simulink model "Transicao"  (R2015b)
settings: Solver=FixedStepAuto  StartTime=0  StopTime=120  FixedStep=sampleTime  RelTol=1e-3
InitFcn:
  | sampleTime = 0.01;
  | Ktd = 0.0526/1000;
  | Kdd = 0.0526/1000;
  | Lb = [0.27 0.27 0.27 0.27];
  | LbAssimetrico  = [0.27 0.27 0.18 0.36];
  | LbTeste  = [0.27 0.27 0.18 0.36];
  | Ixx = 0.0754483;
  | Iyy = 0.13642;
  | Izz = 0.2043333;
  | 
  | IXYZ = [Ixx 0 0; 0 Iyy 0; 0 0 Izz];
  | 
  | areaLateral = [0.0114398 0 0; 0 0.09533687 0; 0 0 0.33];
  | 
  | areaAsa = 0.243;
  | areaProfundor = 0.051;
  | densidadeAr = 1.2;
  | cdArrastoParasita = 1.5;
  | clAviao = 0.825;
  | cdAviao = 0.0743;
  | g = 9.8;
  | massa = 3;
  | velCruzeiro = 15;
  | 
  | inicioTransicao = 40;
  | inicioDesativaAtivacao = 80;
  | 
  | global kroll
  | global kpitch
  | global kyaw
  | 
  | global kx
  | global ky
  | global kz
  | 
  | %Voo em cruzeiro
  | global ku
  | global kzprof
  | global kpitchprof
undefined symbols (not defined in the file or in its folder): DiscIntNeverNeededParam, kpitch, kpitchprof, kroll, ku, kx, kyaw, kz, kzprof
libraries: simulink x17, aerolibwind2 x1
(part 1 of 2)
settings Model: Creator=Avell-G1711  LastModifiedBy=Avell-G1711

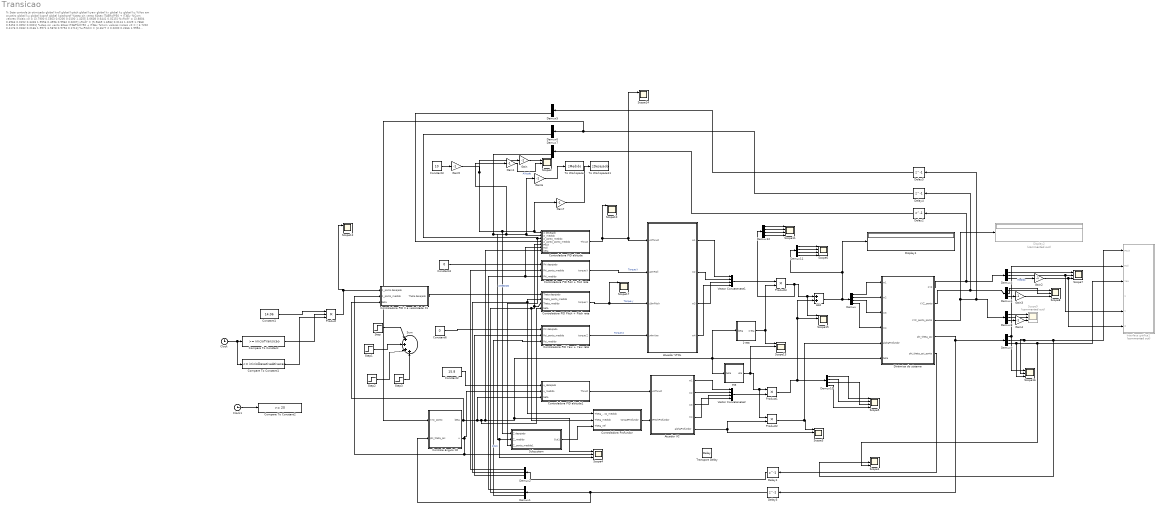
== system Transicao ==
  note: % Seta controle já otimizado
      | global kroll
      | global kpitch
      | global kyaw
      | global kx
      | global ky
      | global kz
      |
      | %Voo em cruzeiro
      | global ku
      | global kzprof
      | global kpitchprof
      |
      | %step sin vento 60sec ITAERoll*50 + ITAEy
      | %Com valores iniciais x0 = [3.7900    0.1663    0.0200    0.0100    1.4255    3.0608    0.6441    0.0215]
      | %xRollY = [3.8804    0.3963    0.0152    0.3328    1.9556    0.4596 0.9962    0.0207]
      | xRollY = [5.5669    1.6582    0.0113    1.2229    1.7868    0.5453    0.0052    0.0001]
      |
      | %step sin vento 60sec ITAEPitch*50 + ITAEx
      | %Com valores iniciais x0 = [ 3.7202    0.4176    0.0182    0.2166    1.9971    3.5878    0.9794    0.1711]
      | %xPitchX = [3.3677    2    0.0200    0.2366    1.9994    0.5776    0.9994    0.0200]
      | %xPitchX = [4.4401    2.8617    0.0114    1.9908    1.9994    4.5196    0.9994    0.0146]
      | %ISExPitchX = [4.0959    0.7473    0.0117    0.0115    2.6735    5.2103    1.9231    0.0301]
      |
      | % VTOL
      | xPitchX = [3.4125    1.4194    0.0110    0.2067    1.8694    3.1439    1.6099    0.0001]
      |
      | %QUASEVTOL mudou apenas o velocidade X pra ajudar na desaceleração
      | xPitchX1 = [3.4125    1.4194    0.0110    0.2067    1.8694    0.6    1.6099    0.0001]
      | %Beta até pi/2.5
      | %xPitchX2 = [8.0000    4.9999    0.0003    2.0000     1.9994    0.5776    0.9994    0.0200]
      |
      | %Beta depois de pi/2.5 (só pra pitch
      | xPitchX2 = [7.1864    4.9121    0.1706    1.1068   1.9994    3.1439    1.6099    0.0001]
      |
      | %Durante VC, foda-se a velocidade em VTOL
      | xPitchX3 = [7.1864    4.9121    0.1706    1.1068   1.9994   0    0    0]
      |
      |
      | %xPitchX2 = [7.1864    4.9121    0.1706    1.1068   1.9994    0    0    0]
      |
      |
      | %beta = 0
      | %xZ = [1.0370    7.9791    1.4905    0.0191    1.2406]
      | xZ = [1.1656    8   3.6063  0   0.6026]
      | %beta = alto
      | xZ2 = [0.1    20    2.5    0    0.5]
      |
      |
      | %Velocidade transição
      | %xu = [3.9966    0.0200    0.0000]
      | %xu = [7.9999    0.0123    1.9988]
      | %xu = [7.9999    0.0123    1.9995]
      | %xu = [15.0000    0.0000    2.2014]
      |
      | %xu 90 graus
      |
      | %xu = [7.9980    0.0015    0.9654]
      | %xu em transicao
      | xu = [10    0.0044    0.0201] %<pi/2.5
      | xu2 = [10    0.0044      5] %>pi/2.5
      |
      |
      |
      | %beta 90 graus
      | %xpitchz = [7.9805    0.0011    0.0210    1.9925    0.0002    0.0360    0.3908    0.0000    0.0000   0.0231    0.0014    0.0263]
      |
      | xpitchz = [9.9883    0.0015    0.0210    7.9750    0.0001    0.0000    0.5    0.0001    0.0000   0.04    0.0051    0.03]
      |
      |
      | kroll.kp = xRollY(1);
      | kroll.kp_ponto = xRollY(2);
      | kroll.kd_ponto = xRollY(3);
      | kroll.ki_ponto = xRollY(4);
      |
      | kpitch.betas = [0   pi/8];
      | kpitch.kp = [xPitchX(1) xPitchX2(1)];
      | kpitch.kp_ponto = [xPitchX(2) xPitchX2(2)];
      | kpitch.kd_ponto = [xPitchX(3) xPitchX2(3)];
      | kpitch.ki_ponto = [xPitchX(4) xPitchX2(4)];
      |
      | kyaw.kp = 2;
      | kyaw.kp_ponto = 2;
      | kyaw.kd_ponto = 0.0134;
      | kyaw.ki_ponto = 2;
      |
      | kx.betas = [pi/3  pi/2.5];
      | kx.kp = xPitchX(5);
      | kx.kp_ponto = [xPitchX1(6)   xPitchX3(6)];
      | kx.kd_ponto =  [xPitchX1(7)   xPitchX3(7)];
      | kx.ki_ponto =  [xPitchX1(8)   xPitchX3(8)];
      |
      | ky.kp = xRollY(5);
      | ky.kp_ponto = xRollY(6);
      | ky.kd_ponto = xRollY(7);
      | ky.ki_ponto = xRollY(8);
      |
      | kz.betas = [0   pi/6];
      | kz.kp = [xZ(1)  xZ2(1)];
      | kz.kp_ponto = [xZ(2)  xZ2(2)];
      | kz.kp_ponto_ponto = [xZ(3)  xZ2(3)];
      | kz.kd_ponto_ponto = [xZ(4)  xZ2(4)];
      | kz.ki_ponto_ponto = [xZ(5)  xZ2(5)];
      |
      | ku.betas = [pi/2.5  pi/2]
      | ku.kp = [xu(1)  xu2(1)];
      | ku.kd = [xu(2)  xu2(2)];
      | ku.ki = [xu(3)  xu2(3)];
      |
      |
      |
      | kpitchprof.kp = xpitchz(1);
      | kpitchprof.kd = xpitchz(2);
      | kpitchprof.ki = xpitchz(3);
      | kpitchprof.kp_ponto = xpitchz(4);
      | kpitchprof.kd_ponto = xpitchz(5);
      | kpitchprof.ki_ponto = xpitchz(6);
      |
      | kzprof.kp = xpitchz(7);
      | kzprof.kd = xpitchz(8);
      | kzprof.ki = xpitchz(9);
      | kzprof.kp_ponto = xpitchz(10);
      | kzprof.kd_ponto = xpitchz(11);
      | kzprof.ki_ponto = xpitchz(12);
      |
      |
      | % global eta
      | % global beta
      | % beta = pi/12;
      | % eta = beta/(pi/2)
      | a=10;
  1-eta : Subsystem
  Add : Sum
  Atuador VC : Subsystem
  Atuador VTOL : Subsystem
  Clock : Clock
  Clock1 : Clock
  Compare To Constant : simulink/Logic and Bit Operations/Compare To Constant  relop=>=  const=inicioTransicao  OutDataTypeStr=boolean
  Compare To Constant1 : simulink/Logic and Bit Operations/Compare To Constant  relop=<=  const=inicioDesativaAtivacao  OutDataTypeStr=boolean
  Compare To Constant2 : simulink/Logic and Bit Operations/Compare To Constant  relop=>=  const=20  OutDataTypeStr=boolean
  Constant1 : Constant  Value=14.06
  Constant2 : Constant  Value=15.8
  Constant3 : Constant  Value=10
  Constant4 : Constant  Value=0
  Constant6 : Constant  Value=0
  Controladora PID Pitch + Pitch rate : Subsystem
  Controladora PID Roll + Roll rate : Subsystem
  Controladora PID X e velocidade X1 : Subsystem
  Controladora PID Yaw + Yaw rate : Subsystem
  Controladora PID altitude : Subsystem
  Controladora PID altitude1 : Subsystem
  Controladora Profundor : Subsystem
  Controle ângulo tilt : Subsystem
  Delay{1..5} (5 alike) : Delay  DelayLength=1  InitialCondition=[0 0 0]
  Demux{,10..12} (4 alike) : Demux
  Demux{1..9} (9 alike) : Demux  Outputs=3
  Dinâmica do sistema : Subsystem
  Display1 : Display
  Display2 : Display  Commented=on
  Gain{,1..7} (8 alike) : Gain  Gain=-1
  Interface gráfica1 : Subsystem  Commented=on  AncestorBlock=vampLib/Interface gráfica
  Product : Product  Inputs=3
  Product1 : Product
  Product2 : Product
  Product3 : Product
  Scope{1..2,4,7..8,12,14,16} (8 alike) : Scope  NumInputPorts=3
  Scope{3,5..6,10..11,13,15,17} (8 alike) : Scope  NumInputPorts=4
  Scope9 : Scope  Commented=on  NumInputPorts=3
  Step : Step  Time=0  After=10  SampleTime=0
  Step1 : Step  Time=20  After=10  SampleTime=0
  Step2 : Step  Time=50  After=-20  SampleTime=0
  Step3 : Step  Time=80  After=10  SampleTime=0
  Subsystem : Subsystem
  Sum : Sum  Inputs=|++++
  To Workspace : ToWorkspace  VariableName=zMedido  SaveFormat=Timeseries  SampleTime=-1
  To Workspace11 : ToWorkspace  VariableName=zDesejado  SaveFormat=Timeseries  SampleTime=-1
  Transport Delay : TransportDelay  DelayTime=20
  Vector Concatenate1 : Concatenate  NumInputs=4
  Vector Concatenate2 : Concatenate  NumInputs=4
  eta : Subsystem
  wires:
  Demux3/1 -> Scope7/1
  Demux3/2 -> Interface gráfica1/5(Y), Scope7/2
  Demux3/3 -> Gain2/1  "Medido"
  Demux4/1 -> Scope8/1
  Demux4/2 -> Scope8/2
  Demux4/3 -> Gain3/1
  Dinâmica do sistema/2(XYZ_ponto) -> Delay4/1, Demux4/1
  Dinâmica do sistema/4(phi_theta_psi) -> Demux9/1, Delay3/1
  Dinâmica do sistema/5(phi_theta_psi_ponto) -> Delay1/1
  Delay1/1 -> Demux2/1
  Demux2/1 -> Controladora PID Roll + Roll rate/2(Phi_ponto_medido)
  Demux2/2 -> Controladora Profundor/1(Theta_ponto_medido), Controladora PID Pitch + Pitch rate/2(Theta_ponto_medido)
  Demux2/3 -> Controladora PID Yaw + Yaw rate/2(Psi_ponto_medido)
  Demux1/1 -> Controladora PID altitude/6(Roll), Controladora PID Roll + Roll rate/3(Phi_medido)
  Demux1/2 -> Controladora Profundor/2(Theta_medido), Controladora PID altitude/5(Pitch), Controladora PID Pitch + Pitch rate/3(Theta_medido)  "Pitch"
  Controladora PID Roll + Roll rate/1(torque X) -> Atuador VTOL/2(u2mRoll)  "Torque X"
  Controladora PID Pitch + Pitch rate/1(torque Y) -> Scope17/1, Atuador VTOL/3(u3mPitch)  "Torque y"
  Controladora PID Yaw + Yaw rate/1(torque Z) -> Atuador VTOL/4(u4mYaw)  "Torque Z"
  Demux7/3 -> Scope4/3, Subsystem/2(Z_medido), Controladora PID altitude/2(Z_medido), Gain6/1, Gain1/1  "ZMEDIDO"
  Dinâmica do sistema/1(XYZ) -> Delay2/1, Demux3/1
  Delay5/1 -> Demux5/1
  Delay4/1 -> Controle ângulo tilt/1(XYZ_ponto), Demux6/1
  Delay2/1 -> Demux7/1
  Demux5/3 -> Controladora PID altitude/4(Z_ponto_ponto_medido)
  Demux6/3 -> Subsystem/3(Z_ponto_medido1), Controladora PID altitude/3(Z_ponto_medido)
  Demux8/1 -> Scope9/1
  Demux8/2 -> Scope9/2
  Demux8/3 -> Gain4/1
  Dinâmica do sistema/3(XYZ_ponto_ponto) -> Display2/1, Demux8/1, Delay5/1
  Gain/1 -> Scope2/1
  Gain1/1 -> Scope2/2  "Alitude"
  Gain2/1 -> Interface gráfica1/6(Z), Scope7/3
  Gain3/1 -> Scope8/3
  Gain4/1 -> Scope9/3
  Demux9/3 -> Scope16/3, Scope1/3, Interface gráfica1/3(Yaw)
  Controladora PID altitude/1(Thrust) -> Scope10/1, Scope14/1, Atuador VTOL/1(u1Thrust)
  Demux1/3 -> Controladora PID Yaw + Yaw rate/3(Psi_medido)
  Gain5/1 -> Subsystem/1(Z desejado), Gain7/1, Controladora PID altitude/1(Z desejado), Gain/1
  Controladora PID altitude1/1(Thrust) -> Atuador VC/1(u1Thrust)
  Atuador VTOL/1(w1) -> Vector Concatenate1/1
  Atuador VTOL/2(w2) -> Vector Concatenate1/2
  Atuador VTOL/3(w3) -> Vector Concatenate1/3
  Atuador VTOL/4(w4) -> Vector Concatenate1/4
  Atuador VC/1(w1) -> Vector Concatenate2/1
  Atuador VC/2(w2) -> Vector Concatenate2/2
  Atuador VC/3(w3) -> Vector Concatenate2/3
  Atuador VC/4(w4) -> Vector Concatenate2/4
  Vector Concatenate2/1 -> Product1/2
  eta/1(eta) -> Scope13/2, Product2/1, Product1/1
  Demux/1 -> Dinâmica do sistema/1(w1)
  Demux/2 -> Dinâmica do sistema/2(w2)
  Demux/3 -> Dinâmica do sistema/3(w3)
  Demux/4 -> Dinâmica do sistema/4(w4)
  Atuador VC/5(alphaProfundor) -> Product2/2, Scope3/2
  Product2/1 -> Dinâmica do sistema/5(alphaProfundor), Scope3/1
  Controle ângulo tilt/1(beta) -> Controladora PID altitude1/3(beta), Controladora PID Pitch + Pitch rate/4(beta), Controladora PID altitude/7(beta), Scope4/1, 1-eta/1(beta), eta/1(beta), Dinâmica do sistema/6(beta), Controladora PID X e velocidade X1/3(beta)
  Controle ângulo tilt/2(u) -> Controladora PID altitude1/2(u_medido), Scope4/2, Controladora PID X e velocidade X1/2(X_ponto_medido)
  Delay3/1 -> Controle ângulo tilt/2(phi_theta_psi), Demux1/1
  Constant4/1 -> Controladora PID Roll + Roll rate/1(Phi desejado)
  Controladora PID X e velocidade X1/1(Theta desejado) -> Controladora PID Pitch + Pitch rate/1(Theta desejado)
  Constant6/1 -> Controladora PID Yaw + Yaw rate/1(Psi desejado)
  Controladora Profundor/1(torqueProfundor) -> Atuador VC/2(tPitchProfundor)
  Demux9/1 -> Scope16/1, Interface gráfica1/2(Roll)
  Subsystem/1(Out1) -> Controladora Profundor/3(Theta_ref)
  1-eta/1(1-eta) -> Product3/2, Scope13/1
  Demux10/1 -> Scope5/1
  Demux10/2 -> Scope5/2
  Demux10/3 -> Scope5/3
  Demux10/4 -> Scope5/4
  Product1/1 -> Add/2, Scope15/2, Demux10/1
  Demux11/1 -> Scope6/1
  Demux11/2 -> Scope6/2
  Demux11/3 -> Scope6/3
  Demux11/4 -> Scope6/4
  Demux12/1 -> Scope11/1
  Demux12/2 -> Scope11/2
  Demux12/3 -> Scope11/3
  Demux12/4 -> Scope11/4
  Product3/1 -> Demux12/1, Scope15/1, Add/1
  Vector Concatenate1/1 -> Product3/1
  Add/1 -> Display1/1, Demux11/1, Demux/1
  Demux9/2 -> Scope16/2, Scope1/2, Interface gráfica1/1(Pitch)
  Clock/1 -> Compare To Constant1/1, Compare To Constant/1
  Compare To Constant/1 -> Product/2
  Compare To Constant1/1 -> Product/3
  Constant1/1 -> Product/1
  Product/1 -> Scope12/1, Controladora PID X e velocidade X1/1(X_ponto desejado)
  Step/1 -> Sum/1
  Step1/1 -> Sum/2
  Step2/1 -> Sum/3
  Step3/1 -> Sum/4
  Clock1/1 -> Compare To Constant2/1
  Gain6/1 -> To Workspace/1
  Gain7/1 -> To Workspace11/1
  Constant2/1 -> Controladora PID altitude1/1(u_desejado)
  Constant3/1 -> Gain5/1

== system Transicao/1-eta ==
  beta : Inport
  Constant : Constant  Value=pi/2
  Constant1 : Constant
  Divide : Product  Inputs=*/
  Sum : Sum  Inputs=|+-
  1-eta : Outport
  wires:
  beta/1 -> Divide/1
  Divide/1 -> Sum/2
  Constant/1 -> Divide/2
  Constant1/1 -> Sum/1
  Sum/1 -> 1-eta/1

== system Transicao/Atuador VC ==
  u1Thrust : Inport
  tPitchProfundor : Inport  Port=2
  Kdd1 : Constant  Value=Kdd
  Ktd1 : Constant  Value=Ktd
  Motor mixer : MATLAB Function  TreatAsAtomicUnit=on
  ib1 : Constant  Value=Lb
  w1 : Outport
  w2 : Outport  Port=2
  w3 : Outport  Port=3
  w4 : Outport  Port=4
  alphaProfundor : Outport  Port=5
  wires:
  tPitchProfundor/1 -> Motor mixer/2(u3mPitch)
  ib1/1 -> Motor mixer/5(lb)
  Motor mixer/2(w2) -> w2/1
  Motor mixer/1(w1) -> w1/1
  u1Thrust/1 -> Motor mixer/1(u1thrust)
  Motor mixer/3(w3) -> w3/1
  Motor mixer/4(w4) -> w4/1
  Ktd1/1 -> Motor mixer/3(ktd)
  Kdd1/1 -> Motor mixer/4(kdd)
  Motor mixer/5(alphaProfundor) -> alphaProfundor/1

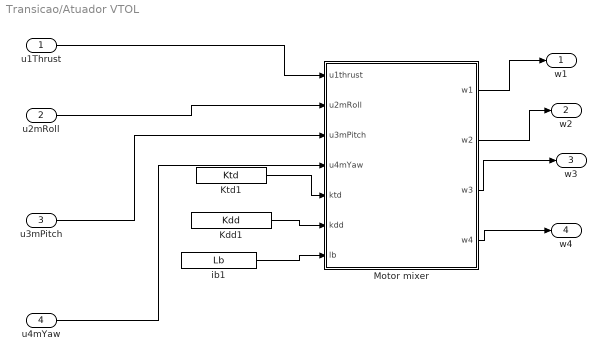
== system Transicao/Atuador VTOL ==
  u1Thrust : Inport
  u2mRoll : Inport  Port=2
  u3mPitch : Inport  Port=3
  u4mYaw : Inport  Port=4
  Kdd1 : Constant  Value=Kdd
  Ktd1 : Constant  Value=Ktd
  Motor mixer : MATLAB Function  TreatAsAtomicUnit=on
  ib1 : Constant  Value=Lb
  w1 : Outport
  w2 : Outport  Port=2
  w3 : Outport  Port=3
  w4 : Outport  Port=4
  wires:
  u3mPitch/1 -> Motor mixer/3(u3mPitch)
  ib1/1 -> Motor mixer/7(lb)
  Motor mixer/2(w2) -> w2/1
  Motor mixer/1(w1) -> w1/1
  u1Thrust/1 -> Motor mixer/1(u1thrust)
  Motor mixer/3(w3) -> w3/1
  Motor mixer/4(w4) -> w4/1
  u4mYaw/1 -> Motor mixer/4(u4mYaw)
  u2mRoll/1 -> Motor mixer/2(u2mRoll)
  Ktd1/1 -> Motor mixer/5(ktd)
  Kdd1/1 -> Motor mixer/6(kdd)

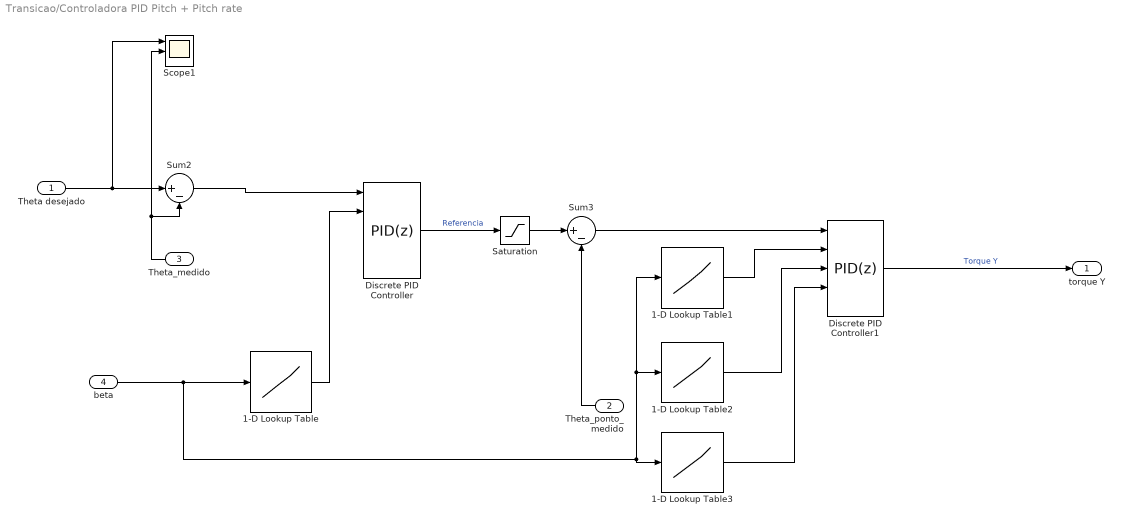
== system Transicao/Controladora PID Pitch + Pitch rate ==
  Theta desejado : Inport
  Theta_ponto_medido : Inport  Port=2
  Theta_medido : Inport  Port=3
  beta : Inport  Port=4
  1-D Lookup Table : Lookup_n-D  NumberOfTableDimensions=1  BreakpointsForDimension1=kpitch.betas  Table=kpitch.kp  ExtrapMethod=Clip  UseLastTableValue=on  InternalRulePriority=Speed  RndMeth=Simplest  InputSameDT=on
  1-D Lookup Table1 : Lookup_n-D  NumberOfTableDimensions=1  BreakpointsForDimension1=kpitch.betas  Table=kpitch.kp_ponto  ExtrapMethod=Clip  UseLastTableValue=on  InternalRulePriority=Speed  RndMeth=Simplest  InputSameDT=on
  1-D Lookup Table2 : Lookup_n-D  NumberOfTableDimensions=1  BreakpointsForDimension1=kpitch.betas  Table=kpitch.ki_ponto  ExtrapMethod=Clip  UseLastTableValue=on  InternalRulePriority=Speed  RndMeth=Simplest  InputSameDT=on
  1-D Lookup Table3 : Lookup_n-D  NumberOfTableDimensions=1  BreakpointsForDimension1=kpitch.betas  Table=kpitch.kd_ponto  ExtrapMethod=Clip  UseLastTableValue=on  InternalRulePriority=Speed  RndMeth=Simplest  InputSameDT=on
  Discrete PID Controller : simulink/Continuous/PID Controller  Controller=PID  TimeDomain=Discrete-time  SampleTime=-1  IntegratorMethod=Forward Euler  FilterMethod=Forward Euler  Form=Parallel  UseFilter=on  ControllerParametersSource=external  P=1  I=1  D=0  N=100  InitialConditionSource=internal  InitialConditionForIntegrator=0  InitialConditionForFilter=0  ExternalReset=none  LimitOutput=off  UpperSaturationLimit=inf  LowerSaturationLimit=-inf  LinearizeAsGain=off  AntiWindupMode=none  Kb=1  TrackingMode=off  Kt=1  PParamMin=[]  PParamMax=[]  IParamMin=[]  IParamMax=[]  DParamMin=[]  DParamMax=[]  NParamMin=[]  NParamMax=[]  KbParamMin=[]  KbParamMax=[]  KtParamMin=[]  KtParamMax=[]  POutMin=[]  POutMax=[]  IOutMin=[]  IOutMax=[]  DOutMin=[]  DOutMax=[]  NOutMin=[]  NOutMax=[]  KbOutMin=[]  KbOutMax=[]  KtOutMin=[]  KtOutMax=[]  IntegratorOutMin=[]  IntegratorOutMax=[]  FilterOutMin=[]  FilterOutMax=[]  SumOutMin=[]  SumOutMax=[]  SumI1OutMin=[]  SumI1OutMax=[]  SumI2OutMin=[]  SumI2OutMax=[]  SumI3OutMin=[]  SumI3OutMax=[]  SumDOutMin=[]  SumDOutMax=[]  SaturationOutMin=[]  SaturationOutMax=[]  IntegratorContinuousStateAttributes=''  IntegratorStateMustResolveToSignalObject=off  IntegratorRTWStateStorageClass=Auto  FilterContinuousStateAttributes=''  FilterStateMustResolveToSignalObject=off  FilterRTWStateStorageClass=Auto  DifferentiatorICPrevScaledInput=0  DifferentiatorOutMin=[]  DifferentiatorOutMax=[]
  Discrete PID Controller1 : simulink/Continuous/PID Controller  Controller=PID  TimeDomain=Discrete-time  SampleTime=-1  IntegratorMethod=Forward Euler  FilterMethod=Forward Euler  Form=Parallel  UseFilter=on  ControllerParametersSource=external  P=1  I=1  D=0  N=100  InitialConditionSource=internal  InitialConditionForIntegrator=0  InitialConditionForFilter=0  ExternalReset=none  LimitOutput=off  UpperSaturationLimit=inf  LowerSaturationLimit=-inf  LinearizeAsGain=off  AntiWindupMode=none  Kb=1  TrackingMode=off  Kt=1  PParamMin=[]  PParamMax=[]  IParamMin=[]  IParamMax=[]  DParamMin=[]  DParamMax=[]  NParamMin=[]  NParamMax=[]  KbParamMin=[]  KbParamMax=[]  KtParamMin=[]  KtParamMax=[]  POutMin=[]  POutMax=[]  IOutMin=[]  IOutMax=[]  DOutMin=[]  DOutMax=[]  NOutMin=[]  NOutMax=[]  KbOutMin=[]  KbOutMax=[]  KtOutMin=[]  KtOutMax=[]  IntegratorOutMin=[]  IntegratorOutMax=[]  FilterOutMin=[]  FilterOutMax=[]  SumOutMin=[]  SumOutMax=[]  SumI1OutMin=[]  SumI1OutMax=[]  SumI2OutMin=[]  SumI2OutMax=[]  SumI3OutMin=[]  SumI3OutMax=[]  SumDOutMin=[]  SumDOutMax=[]  SaturationOutMin=[]  SaturationOutMax=[]  IntegratorContinuousStateAttributes=''  IntegratorStateMustResolveToSignalObject=off  IntegratorRTWStateStorageClass=Auto  FilterContinuousStateAttributes=''  FilterStateMustResolveToSignalObject=off  FilterRTWStateStorageClass=Auto  DifferentiatorICPrevScaledInput=0  DifferentiatorOutMin=[]  DifferentiatorOutMax=[]
  Saturation : Saturate  UpperLimit=pi  LowerLimit=-pi
  Scope1 : Scope  NumInputPorts=3
  Sum2 : Sum  Inputs=|+-
  Sum3 : Sum  Inputs=|+-
  torque Y : Outport
  wires:
  Theta_ponto_medido/1 -> Sum3/2
  Theta_medido/1 -> Scope1/2, Sum2/2
  Sum2/1 -> Discrete PID Controller/1
  Sum3/1 -> Discrete PID Controller1/1
  Theta desejado/1 -> Scope1/1, Sum2/1
  Discrete PID Controller/1 -> Saturation/1  "Referencia"
  Discrete PID Controller1/1 -> torque Y/1  "Torque Y"
  beta/1 -> 1-D Lookup Table1/1, 1-D Lookup Table2/1, 1-D Lookup Table3/1, 1-D Lookup Table/1
  1-D Lookup Table/1 -> Discrete PID Controller/2
  1-D Lookup Table1/1 -> Discrete PID Controller1/2
  1-D Lookup Table2/1 -> Discrete PID Controller1/3
  1-D Lookup Table3/1 -> Discrete PID Controller1/4
  Saturation/1 -> Sum3/1

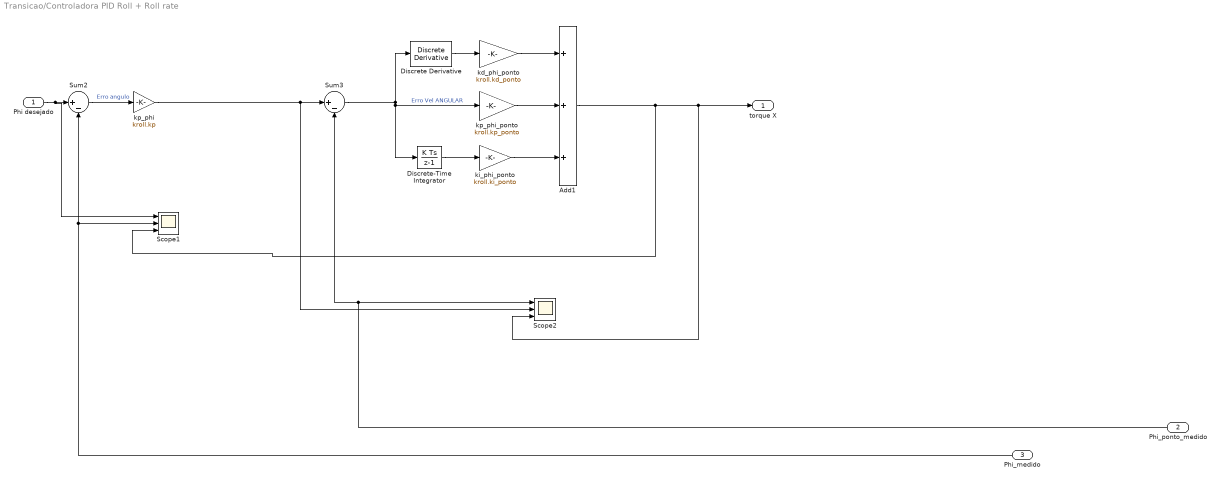
== system Transicao/Controladora PID Roll + Roll rate ==
  Phi desejado : Inport
  Phi_ponto_medido : Inport  Port=2
  Phi_medido : Inport  Port=3
  Add1 : Sum  Inputs=+++
  Discrete Derivative : simulink/Discrete/Discrete Derivative  gainval=1.0  ICPrevScaledInput=0.0  InputProcessing=Inherited  OutMin=[]  OutMax=[]  OutDataType=fixdt(1, 16)  OutScaling=2^-10  DoSatur=off
  Discrete-Time Integrator : DiscreteIntegrator  InitialConditionSetting=State (most efficient)  SampleTime=-1  ICPrevOutput=DiscIntNeverNeededParam  ICPrevScaledInput=DiscIntNeverNeededParam
  Scope1 : Scope  NumInputPorts=3
  Scope2 : Scope  NumInputPorts=3
  Sum2 : Sum  Inputs=|+-
  Sum3 : Sum  Inputs=|+-
  kd_phi_ponto : Gain  Gain=kroll.kd_ponto
  ki_phi_ponto : Gain  Gain=kroll.ki_ponto
  kp_phi : Gain  Gain=kroll.kp
  kp_phi_ponto : Gain  Gain=kroll.kp_ponto
  torque X : Outport
  wires:
  Phi_ponto_medido/1 -> Sum3/2, Scope2/1
  Discrete-Time Integrator/1 -> ki_phi_ponto/1
  Add1/1 -> Scope1/3, Scope2/3, torque X/1
  kd_phi_ponto/1 -> Add1/1
  Sum2/1 -> kp_phi/1  "Erro angulo"
  ki_phi_ponto/1 -> Add1/3
  Discrete Derivative/1 -> kd_phi_ponto/1
  kp_phi_ponto/1 -> Add1/2
  Phi desejado/1 -> Scope1/1, Sum2/1
  Sum3/1 -> Discrete-Time Integrator/1, kp_phi_ponto/1, Discrete Derivative/1  "Erro Vel ANGULAR"
  Phi_medido/1 -> Scope1/2, Sum2/2
  kp_phi/1 -> Scope2/2, Sum3/1

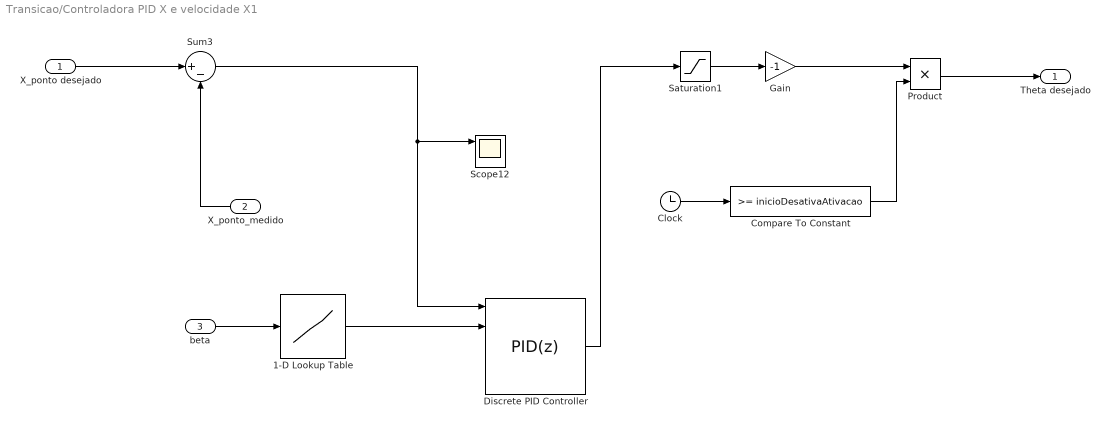
== system Transicao/Controladora PID X e velocidade X1 ==
  X_ponto desejado : Inport
  X_ponto_medido : Inport  Port=2
  beta : Inport  Port=3
  1-D Lookup Table : Lookup_n-D  NumberOfTableDimensions=1  BreakpointsForDimension1=kx.betas  Table=kx.kp_ponto  ExtrapMethod=Clip  UseLastTableValue=on  InternalRulePriority=Speed  RndMeth=Simplest  InputSameDT=on
  Clock : Clock
  Compare To Constant : simulink/Logic and Bit Operations/Compare To Constant  relop=>=  const=inicioDesativaAtivacao  OutDataTypeStr=boolean
  Discrete PID Controller : simulink/Continuous/PID Controller  Controller=PID  TimeDomain=Discrete-time  SampleTime=-1  IntegratorMethod=Forward Euler  FilterMethod=Forward Euler  Form=Parallel  UseFilter=on  ControllerParametersSource=external  P=1  I=1  D=0  N=100  InitialConditionSource=internal  InitialConditionForIntegrator=0  InitialConditionForFilter=0  ExternalReset=none  LimitOutput=off  UpperSaturationLimit=inf  LowerSaturationLimit=-inf  LinearizeAsGain=off  AntiWindupMode=none  Kb=1  TrackingMode=off  Kt=1  PParamMin=[]  PParamMax=[]  IParamMin=[]  IParamMax=[]  DParamMin=[]  DParamMax=[]  NParamMin=[]  NParamMax=[]  KbParamMin=[]  KbParamMax=[]  KtParamMin=[]  KtParamMax=[]  POutMin=[]  POutMax=[]  IOutMin=[]  IOutMax=[]  DOutMin=[]  DOutMax=[]  NOutMin=[]  NOutMax=[]  KbOutMin=[]  KbOutMax=[]  KtOutMin=[]  KtOutMax=[]  IntegratorOutMin=[]  IntegratorOutMax=[]  FilterOutMin=[]  FilterOutMax=[]  SumOutMin=[]  SumOutMax=[]  SumI1OutMin=[]  SumI1OutMax=[]  SumI2OutMin=[]  SumI2OutMax=[]  SumI3OutMin=[]  SumI3OutMax=[]  SumDOutMin=[]  SumDOutMax=[]  SaturationOutMin=[]  SaturationOutMax=[]  IntegratorContinuousStateAttributes=''  IntegratorStateMustResolveToSignalObject=off  IntegratorRTWStateStorageClass=Auto  FilterContinuousStateAttributes=''  FilterStateMustResolveToSignalObject=off  FilterRTWStateStorageClass=Auto  DifferentiatorICPrevScaledInput=0  DifferentiatorOutMin=[]  DifferentiatorOutMax=[]
  Gain : Gain  Gain=-1
  Product : Product
  Saturation1 : Saturate  UpperLimit=pi/4  LowerLimit=-pi/4  LinearizeAsGain=off
  Scope12 : Scope  NumInputPorts=3
  Sum3 : Sum  Inputs=|+-
  Theta desejado : Outport
  wires:
  X_ponto_medido/1 -> Sum3/2
  Discrete PID Controller/1 -> Saturation1/1
  Saturation1/1 -> Gain/1
  Clock/1 -> Compare To Constant/1
  Gain/1 -> Product/1
  Compare To Constant/1 -> Product/2
  Product/1 -> Theta desejado/1
  1-D Lookup Table/1 -> Discrete PID Controller/2
  beta/1 -> 1-D Lookup Table/1
  Sum3/1 -> Scope12/1, Discrete PID Controller/1
  X_ponto desejado/1 -> Sum3/1

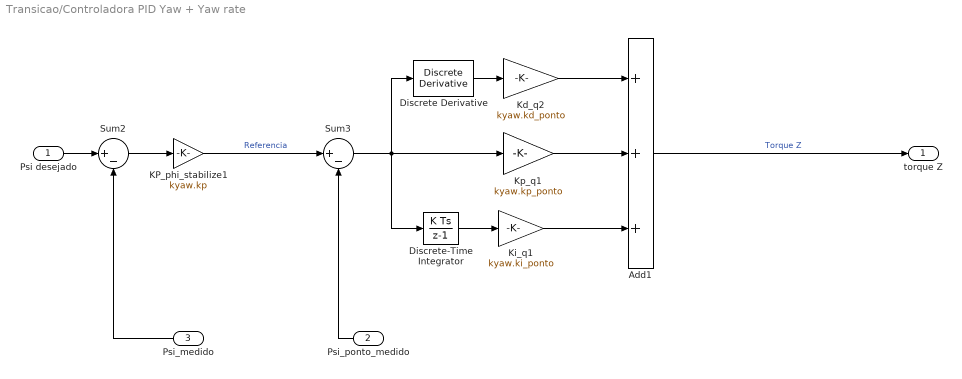
== system Transicao/Controladora PID Yaw + Yaw rate ==
  Psi desejado : Inport
  Psi_ponto_medido : Inport  Port=2
  Psi_medido : Inport  Port=3
  Add1 : Sum  Inputs=+++
  Discrete Derivative : simulink/Discrete/Discrete Derivative  gainval=1.0  ICPrevScaledInput=0.0  InputProcessing=Inherited  OutMin=[]  OutMax=[]  OutDataType=fixdt(1, 16)  OutScaling=2^-10  DoSatur=off
  Discrete-Time Integrator : DiscreteIntegrator  InitialConditionSetting=State (most efficient)  SampleTime=-1  ICPrevOutput=DiscIntNeverNeededParam  ICPrevScaledInput=DiscIntNeverNeededParam
  KP_phi_stabilize1 : Gain  Gain=kyaw.kp
  Kd_q2 : Gain  Gain=kyaw.kd_ponto
  Ki_q1 : Gain  Gain=kyaw.ki_ponto
  Kp_q1 : Gain  Gain=kyaw.kp_ponto
  Sum2 : Sum  Inputs=|+-
  Sum3 : Sum  Inputs=|+-
  torque Z : Outport
  wires:
  Psi_ponto_medido/1 -> Sum3/2
  Discrete-Time Integrator/1 -> Ki_q1/1
  Psi_medido/1 -> Sum2/2
  Kd_q2/1 -> Add1/1
  Sum2/1 -> KP_phi_stabilize1/1
  Ki_q1/1 -> Add1/3
  Discrete Derivative/1 -> Kd_q2/1
  Sum3/1 -> Discrete Derivative/1, Discrete-Time Integrator/1, Kp_q1/1
  Kp_q1/1 -> Add1/2
  Psi desejado/1 -> Sum2/1
  KP_phi_stabilize1/1 -> Sum3/1  "Referencia"
  Add1/1 -> torque Z/1  "Torque Z"

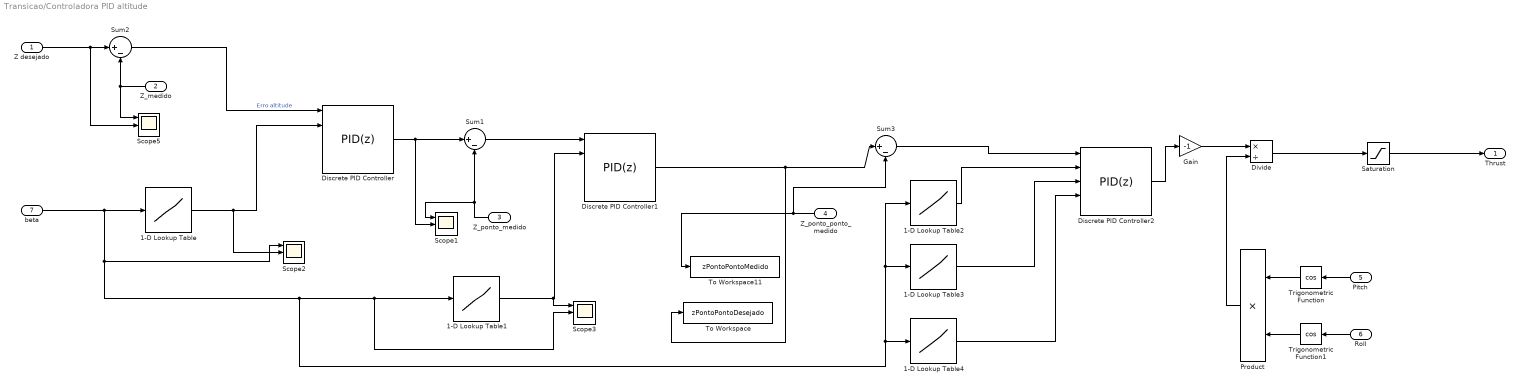
== system Transicao/Controladora PID altitude ==
  Z desejado : Inport
  Z_medido : Inport  Port=2
  Z_ponto_medido : Inport  Port=3
  Z_ponto_ponto_medido : Inport  Port=4
  Pitch : Inport  Port=5
  Roll : Inport  Port=6
  beta : Inport  Port=7
  1-D Lookup Table : Lookup_n-D  NumberOfTableDimensions=1  BreakpointsForDimension1=kz.betas  Table=kz.kp  ExtrapMethod=Clip  UseLastTableValue=on  InternalRulePriority=Speed  RndMeth=Simplest  InputSameDT=on
  1-D Lookup Table1 : Lookup_n-D  NumberOfTableDimensions=1  BreakpointsForDimension1=kz.betas  Table=kz.kp_ponto  ExtrapMethod=Clip  UseLastTableValue=on  InternalRulePriority=Speed  RndMeth=Simplest  InputSameDT=on
  1-D Lookup Table2 : Lookup_n-D  NumberOfTableDimensions=1  BreakpointsForDimension1=kz.betas  Table=kz.kp_ponto_ponto  ExtrapMethod=Clip  UseLastTableValue=on  InternalRulePriority=Speed  RndMeth=Simplest  InputSameDT=on
  1-D Lookup Table3 : Lookup_n-D  NumberOfTableDimensions=1  BreakpointsForDimension1=kz.betas  Table=kz.ki_ponto_ponto  ExtrapMethod=Clip  UseLastTableValue=on  InternalRulePriority=Speed  RndMeth=Simplest  InputSameDT=on
  1-D Lookup Table4 : Lookup_n-D  NumberOfTableDimensions=1  BreakpointsForDimension1=kz.betas  Table=kz.kd_ponto_ponto  ExtrapMethod=Clip  UseLastTableValue=on  InternalRulePriority=Speed  RndMeth=Simplest  InputSameDT=on
  Discrete PID Controller : simulink/Continuous/PID Controller  Controller=PID  TimeDomain=Discrete-time  SampleTime=-1  IntegratorMethod=Forward Euler  FilterMethod=Forward Euler  Form=Parallel  UseFilter=on  ControllerParametersSource=external  P=1  I=1  D=0  N=100  InitialConditionSource=internal  InitialConditionForIntegrator=0  InitialConditionForFilter=0  ExternalReset=none  LimitOutput=off  UpperSaturationLimit=inf  LowerSaturationLimit=-inf  LinearizeAsGain=off  AntiWindupMode=none  Kb=1  TrackingMode=off  Kt=1  PParamMin=[]  PParamMax=[]  IParamMin=[]  IParamMax=[]  DParamMin=[]  DParamMax=[]  NParamMin=[]  NParamMax=[]  KbParamMin=[]  KbParamMax=[]  KtParamMin=[]  KtParamMax=[]  POutMin=[]  POutMax=[]  IOutMin=[]  IOutMax=[]  DOutMin=[]  DOutMax=[]  NOutMin=[]  NOutMax=[]  KbOutMin=[]  KbOutMax=[]  KtOutMin=[]  KtOutMax=[]  IntegratorOutMin=[]  IntegratorOutMax=[]  FilterOutMin=[]  FilterOutMax=[]  SumOutMin=[]  SumOutMax=[]  SumI1OutMin=[]  SumI1OutMax=[]  SumI2OutMin=[]  SumI2OutMax=[]  SumI3OutMin=[]  SumI3OutMax=[]  SumDOutMin=[]  SumDOutMax=[]  SaturationOutMin=[]  SaturationOutMax=[]  IntegratorContinuousStateAttributes=''  IntegratorStateMustResolveToSignalObject=off  IntegratorRTWStateStorageClass=Auto  FilterContinuousStateAttributes=''  FilterStateMustResolveToSignalObject=off  FilterRTWStateStorageClass=Auto  DifferentiatorICPrevScaledInput=0  DifferentiatorOutMin=[]  DifferentiatorOutMax=[]
  Discrete PID Controller1 : simulink/Continuous/PID Controller  Controller=PID  TimeDomain=Discrete-time  SampleTime=-1  IntegratorMethod=Forward Euler  FilterMethod=Forward Euler  Form=Parallel  UseFilter=on  ControllerParametersSource=external  P=1  I=1  D=0  N=100  InitialConditionSource=internal  InitialConditionForIntegrator=0  InitialConditionForFilter=0  ExternalReset=none  LimitOutput=off  UpperSaturationLimit=inf  LowerSaturationLimit=-inf  LinearizeAsGain=off  AntiWindupMode=none  Kb=1  TrackingMode=off  Kt=1  PParamMin=[]  PParamMax=[]  IParamMin=[]  IParamMax=[]  DParamMin=[]  DParamMax=[]  NParamMin=[]  NParamMax=[]  KbParamMin=[]  KbParamMax=[]  KtParamMin=[]  KtParamMax=[]  POutMin=[]  POutMax=[]  IOutMin=[]  IOutMax=[]  DOutMin=[]  DOutMax=[]  NOutMin=[]  NOutMax=[]  KbOutMin=[]  KbOutMax=[]  KtOutMin=[]  KtOutMax=[]  IntegratorOutMin=[]  IntegratorOutMax=[]  FilterOutMin=[]  FilterOutMax=[]  SumOutMin=[]  SumOutMax=[]  SumI1OutMin=[]  SumI1OutMax=[]  SumI2OutMin=[]  SumI2OutMax=[]  SumI3OutMin=[]  SumI3OutMax=[]  SumDOutMin=[]  SumDOutMax=[]  SaturationOutMin=[]  SaturationOutMax=[]  IntegratorContinuousStateAttributes=''  IntegratorStateMustResolveToSignalObject=off  IntegratorRTWStateStorageClass=Auto  FilterContinuousStateAttributes=''  FilterStateMustResolveToSignalObject=off  FilterRTWStateStorageClass=Auto  DifferentiatorICPrevScaledInput=0  DifferentiatorOutMin=[]  DifferentiatorOutMax=[]
  Discrete PID Controller2 : simulink/Continuous/PID Controller  Controller=PID  TimeDomain=Discrete-time  SampleTime=-1  IntegratorMethod=Forward Euler  FilterMethod=Forward Euler  Form=Parallel  UseFilter=on  ControllerParametersSource=external  P=1  I=1  D=0  N=100  InitialConditionSource=internal  InitialConditionForIntegrator=0  InitialConditionForFilter=0  ExternalReset=none  LimitOutput=off  UpperSaturationLimit=inf  LowerSaturationLimit=-inf  LinearizeAsGain=off  AntiWindupMode=none  Kb=1  TrackingMode=off  Kt=1  PParamMin=[]  PParamMax=[]  IParamMin=[]  IParamMax=[]  DParamMin=[]  DParamMax=[]  NParamMin=[]  NParamMax=[]  KbParamMin=[]  KbParamMax=[]  KtParamMin=[]  KtParamMax=[]  POutMin=[]  POutMax=[]  IOutMin=[]  IOutMax=[]  DOutMin=[]  DOutMax=[]  NOutMin=[]  NOutMax=[]  KbOutMin=[]  KbOutMax=[]  KtOutMin=[]  KtOutMax=[]  IntegratorOutMin=[]  IntegratorOutMax=[]  FilterOutMin=[]  FilterOutMax=[]  SumOutMin=[]  SumOutMax=[]  SumI1OutMin=[]  SumI1OutMax=[]  SumI2OutMin=[]  SumI2OutMax=[]  SumI3OutMin=[]  SumI3OutMax=[]  SumDOutMin=[]  SumDOutMax=[]  SaturationOutMin=[]  SaturationOutMax=[]  IntegratorContinuousStateAttributes=''  IntegratorStateMustResolveToSignalObject=off  IntegratorRTWStateStorageClass=Auto  FilterContinuousStateAttributes=''  FilterStateMustResolveToSignalObject=off  FilterRTWStateStorageClass=Auto  DifferentiatorICPrevScaledInput=0  DifferentiatorOutMin=[]  DifferentiatorOutMax=[]
  Divide : Product  Inputs=*/
  Gain : Gain  Gain=-1
  Product : Product
  Saturation : Saturate  UpperLimit=53  LowerLimit=0
  Scope{1..3,5} (4 alike) : Scope  NumInputPorts=3
  Sum1 : Sum  Inputs=|+-
  Sum2 : Sum  Inputs=|+-
  Sum3 : Sum  Inputs=|+-
  To Workspace : ToWorkspace  VariableName=zPontoPontoDesejado  SaveFormat=Timeseries  SampleTime=-1
  To Workspace11 : ToWorkspace  VariableName=zPontoPontoMedido  SaveFormat=Timeseries  SampleTime=-1
  Trigonometric Function : Trigonometry  Operator=cos
  Trigonometric Function1 : Trigonometry  Operator=cos
  Thrust : Outport
  wires:
  Sum2/1 -> Discrete PID Controller/1  "Erro altitude"
  Z desejado/1 -> Scope5/2, Sum2/1
  Z_medido/1 -> Scope5/1, Sum2/2
  Z_ponto_medido/1 -> Scope1/1, Sum1/2
  Discrete PID Controller/1 -> Sum1/1, Scope1/2
  Sum1/1 -> Discrete PID Controller1/1
  Discrete PID Controller1/1 -> Sum3/1, To Workspace/1
  Z_ponto_ponto_medido/1 -> To Workspace11/1, Sum3/2
  Sum3/1 -> Discrete PID Controller2/1
  Pitch/1 -> Trigonometric Function/1
  Roll/1 -> Trigonometric Function1/1
  Product/1 -> Divide/2
  Discrete PID Controller2/1 -> Gain/1
  Trigonometric Function/1 -> Product/1
  Trigonometric Function1/1 -> Product/2
  Gain/1 -> Divide/1
  Saturation/1 -> Thrust/1
  Divide/1 -> Saturation/1
  1-D Lookup Table/1 -> Scope2/2, Discrete PID Controller/2
  1-D Lookup Table1/1 -> Scope3/1, Discrete PID Controller1/2
  1-D Lookup Table2/1 -> Discrete PID Controller2/2
  1-D Lookup Table3/1 -> Discrete PID Controller2/3
  1-D Lookup Table4/1 -> Discrete PID Controller2/4
  beta/1 -> Scope2/1, 1-D Lookup Table4/1, 1-D Lookup Table3/1, 1-D Lookup Table2/1, Scope3/2, 1-D Lookup Table1/1, 1-D Lookup Table/1

== system Transicao/Controladora PID altitude1 ==
  u_desejado : Inport
  u_medido : Inport  Port=2
  beta : Inport  Port=3
  1-D Lookup Table : Lookup_n-D  NumberOfTableDimensions=1  BreakpointsForDimension1=ku.betas  Table=ku.kp  ExtrapMethod=Clip  UseLastTableValue=on  InternalRulePriority=Speed  RndMeth=Simplest  InputSameDT=on
  1-D Lookup Table1 : Lookup_n-D  NumberOfTableDimensions=1  BreakpointsForDimension1=ku.betas  Table=ku.ki  ExtrapMethod=Clip  UseLastTableValue=on  InternalRulePriority=Speed  RndMeth=Simplest  InputSameDT=on
  1-D Lookup Table2 : Lookup_n-D  NumberOfTableDimensions=1  BreakpointsForDimension1=ku.betas  Table=ku.kd  ExtrapMethod=Clip  UseLastTableValue=on  InternalRulePriority=Speed  RndMeth=Simplest  InputSameDT=on
  Discrete PID Controller : simulink/Continuous/PID Controller  Controller=PID  TimeDomain=Discrete-time  SampleTime=-1  IntegratorMethod=Forward Euler  FilterMethod=Forward Euler  Form=Parallel  UseFilter=on  ControllerParametersSource=external  P=1  I=1  D=0  N=100  InitialConditionSource=internal  InitialConditionForIntegrator=0  InitialConditionForFilter=0  ExternalReset=none  LimitOutput=off  UpperSaturationLimit=inf  LowerSaturationLimit=-inf  LinearizeAsGain=off  AntiWindupMode=none  Kb=1  TrackingMode=off  Kt=1  PParamMin=[]  PParamMax=[]  IParamMin=[]  IParamMax=[]  DParamMin=[]  DParamMax=[]  NParamMin=[]  NParamMax=[]  KbParamMin=[]  KbParamMax=[]  KtParamMin=[]  KtParamMax=[]  POutMin=[]  POutMax=[]  IOutMin=[]  IOutMax=[]  DOutMin=[]  DOutMax=[]  NOutMin=[]  NOutMax=[]  KbOutMin=[]  KbOutMax=[]  KtOutMin=[]  KtOutMax=[]  IntegratorOutMin=[]  IntegratorOutMax=[]  FilterOutMin=[]  FilterOutMax=[]  SumOutMin=[]  SumOutMax=[]  SumI1OutMin=[]  SumI1OutMax=[]  SumI2OutMin=[]  SumI2OutMax=[]  SumI3OutMin=[]  SumI3OutMax=[]  SumDOutMin=[]  SumDOutMax=[]  SaturationOutMin=[]  SaturationOutMax=[]  IntegratorContinuousStateAttributes=''  IntegratorStateMustResolveToSignalObject=off  IntegratorRTWStateStorageClass=Auto  FilterContinuousStateAttributes=''  FilterStateMustResolveToSignalObject=off  FilterRTWStateStorageClass=Auto  DifferentiatorICPrevScaledInput=0  DifferentiatorOutMin=[]  DifferentiatorOutMax=[]
  Scope1 : Scope  NumInputPorts=3
  Sum3 : Sum  Inputs=|+-
  To Workspace1 : ToWorkspace  VariableName=uDesejado  SaveFormat=Timeseries  SampleTime=-1
  To Workspace2 : ToWorkspace  VariableName=uMedido  SaveFormat=Timeseries  SampleTime=-1
  Thrust : Outport
  wires:
  u_desejado/1 -> Scope1/1, To Workspace1/1, Sum3/1
  u_medido/1 -> Sum3/2, To Workspace2/1, Scope1/2
  Discrete PID Controller/1 -> Thrust/1
  1-D Lookup Table/1 -> Discrete PID Controller/2
  1-D Lookup Table1/1 -> Discrete PID Controller/3
  1-D Lookup Table2/1 -> Discrete PID Controller/4
  Sum3/1 -> Discrete PID Controller/1
  beta/1 -> 1-D Lookup Table2/1, 1-D Lookup Table1/1, 1-D Lookup Table/1

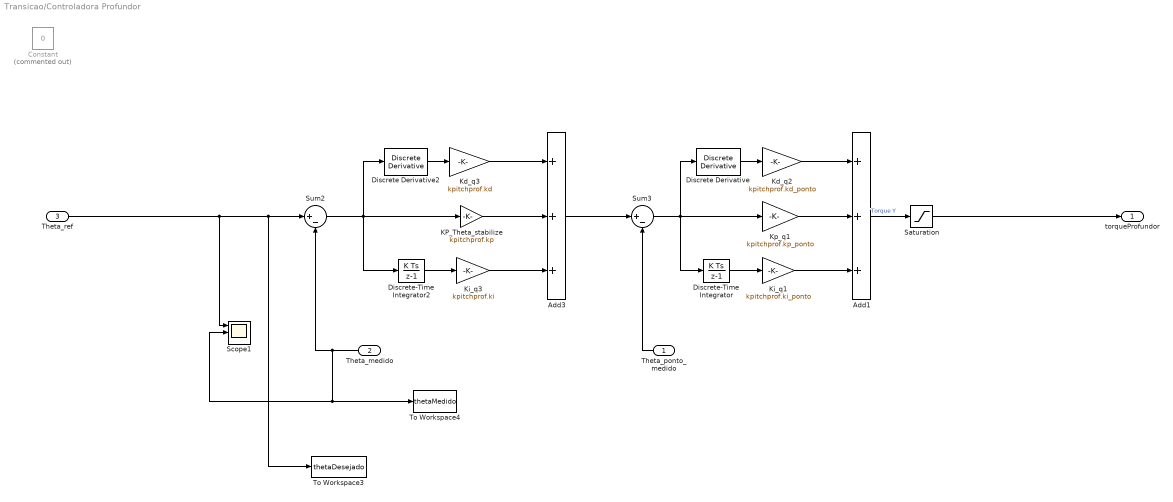
== system Transicao/Controladora Profundor ==
  Theta_ponto_medido : Inport
  Theta_medido : Inport  Port=2
  Theta_ref : Inport  Port=3
  Add1 : Sum  Inputs=+++
  Add3 : Sum  Inputs=+++
  Constant : Constant  Commented=on  Value=0
  Discrete Derivative : simulink/Discrete/Discrete Derivative  gainval=1.0  ICPrevScaledInput=0.0  InputProcessing=Inherited  OutMin=[]  OutMax=[]  OutDataType=fixdt(1, 16)  OutScaling=2^-10  DoSatur=off
  Discrete Derivative2 : simulink/Discrete/Discrete Derivative  gainval=1.0  ICPrevScaledInput=0.0  InputProcessing=Inherited  OutMin=[]  OutMax=[]  OutDataType=fixdt(1, 16)  OutScaling=2^-10  DoSatur=off
  Discrete-Time Integrator : DiscreteIntegrator  InitialConditionSetting=State (most efficient)  SampleTime=-1  ICPrevOutput=DiscIntNeverNeededParam  ICPrevScaledInput=DiscIntNeverNeededParam
  Discrete-Time Integrator2 : DiscreteIntegrator  InitialConditionSetting=State (most efficient)  SampleTime=-1  ICPrevOutput=DiscIntNeverNeededParam  ICPrevScaledInput=DiscIntNeverNeededParam
  KP_Theta_stabilize : Gain  Gain=kpitchprof.kp
  Kd_q2 : Gain  Gain=kpitchprof.kd_ponto
  Kd_q3 : Gain  Gain=kpitchprof.kd
  Ki_q1 : Gain  Gain=kpitchprof.ki_ponto
  Ki_q3 : Gain  Gain=kpitchprof.ki
  Kp_q1 : Gain  Gain=kpitchprof.kp_ponto
  Saturation : Saturate  UpperLimit=2  LowerLimit=-2  LinearizeAsGain=off
  Scope1 : Scope  NumInputPorts=3
  Sum2 : Sum  Inputs=|+-
  Sum3 : Sum  Inputs=|+-
  To Workspace3 : ToWorkspace  VariableName=thetaDesejado  SaveFormat=Timeseries  SampleTime=-1
  To Workspace4 : ToWorkspace  VariableName=thetaMedido  SaveFormat=Timeseries  SampleTime=-1
  torqueProfundor : Outport
  wires:
  Theta_ponto_medido/1 -> Sum3/2
  Discrete-Time Integrator/1 -> Ki_q1/1
  Theta_medido/1 -> To Workspace4/1, Scope1/2, Sum2/2
  Kd_q2/1 -> Add1/1
  Ki_q1/1 -> Add1/3
  Discrete Derivative/1 -> Kd_q2/1
  Sum3/1 -> Discrete Derivative/1, Discrete-Time Integrator/1, Kp_q1/1
  Kp_q1/1 -> Add1/2
  Add1/1 -> Saturation/1  "Torque Y"
  Kd_q3/1 -> Add3/1
  Discrete Derivative2/1 -> Kd_q3/1
  Sum2/1 -> Discrete-Time Integrator2/1, KP_Theta_stabilize/1, Discrete Derivative2/1
  Discrete-Time Integrator2/1 -> Ki_q3/1
  Ki_q3/1 -> Add3/3
  KP_Theta_stabilize/1 -> Add3/2
  Add3/1 -> Sum3/1
  Saturation/1 -> torqueProfundor/1
  Theta_ref/1 -> Scope1/1, To Workspace3/1, Sum2/1

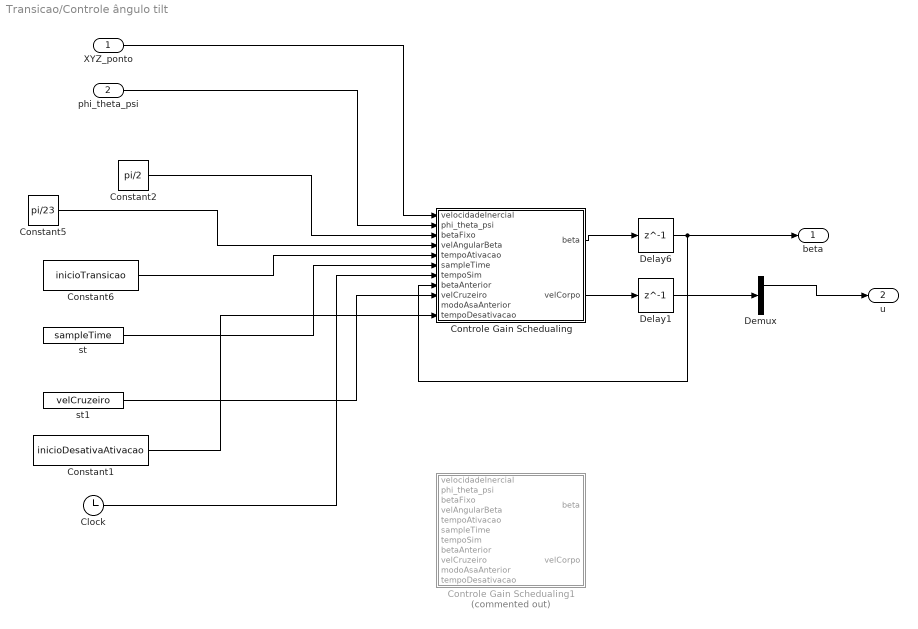
== system Transicao/Controle ângulo tilt ==
  XYZ_ponto : Inport
  phi_theta_psi : Inport  Port=2
  Clock : Clock
  Constant1 : Constant  Value=inicioDesativaAtivacao
  Constant2 : Constant  Value=pi/2
  Constant5 : Constant  Value=pi/23
  Constant6 : Constant  Value=inicioTransicao
  Controle Gain Schedualing : MATLAB Function  TreatAsAtomicUnit=on
  Controle Gain Schedualing1 : MATLAB Function  Commented=on  TreatAsAtomicUnit=on
  Delay1 : Delay  DelayLength=1  InitialCondition=0
  Delay6 : Delay  DelayLength=1  InitialCondition=0
  Demux : Demux  Outputs=3
  st : Constant  Value=sampleTime
  st1 : Constant  Value=velCruzeiro
  beta : Outport
  u : Outport  Port=2
  wires:
  st/1 -> Controle Gain Schedualing/6(sampleTime)
  Constant2/1 -> Controle Gain Schedualing/3(betaFixo)
  Constant5/1 -> Controle Gain Schedualing/4(velAngularBeta)
  XYZ_ponto/1 -> Controle Gain Schedualing/1(velocidadeInercial)
  phi_theta_psi/1 -> Controle Gain Schedualing/2(phi_theta_psi)
  Controle Gain Schedualing/1(beta) -> Delay6/1
  Clock/1 -> Controle Gain Schedualing/7(tempoSim)
  st1/1 -> Controle Gain Schedualing/9(velCruzeiro)
  Constant6/1 -> Controle Gain Schedualing/5(tempoAtivacao)
  Controle Gain Schedualing/2(velCorpo) -> Delay1/1
  Delay1/1 -> Demux/1
  Demux/1 -> u/1
  Constant1/1 -> Controle Gain Schedualing/11(tempoDesativacao)
  Delay6/1 -> beta/1, Controle Gain Schedualing/8(betaAnterior)

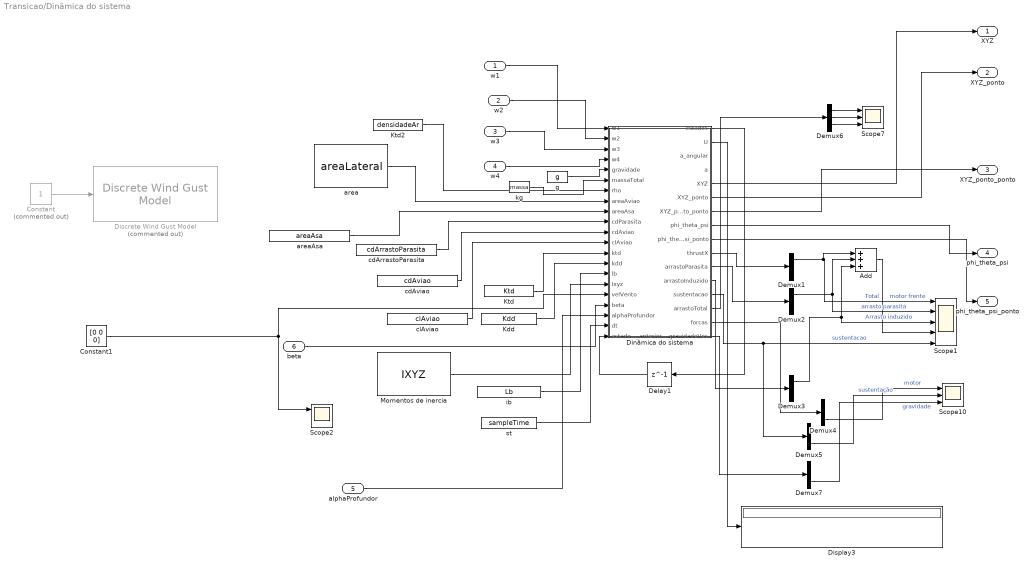
== system Transicao/Dinâmica do sistema ==
  w1 : Inport
  w2 : Inport  Port=2
  w3 : Inport  Port=3
  w4 : Inport  Port=4
  alphaProfundor : Inport  Port=5
  beta : Inport  Port=6
  Add : Sum  Inputs=+++
  Constant : Constant  Commented=on
  Constant1 : Constant  Value=[0 0 0]
  Delay1 : Delay  DelayLength=1  InitialCondition=[0 0 0 0;0 0 0 0;-10 0 0 0]
  Demux{1..7} (7 alike) : Demux  Outputs=3
  Dinâmica do sistema : MATLAB Function  TreatAsAtomicUnit=on
  Discrete Wind Gust Model : aerolibwind2/Discrete Wind Gust Model  Commented=on  units=Metric (MKS)  Gx=on  Gy=on  Gz=on  t_0=40  d_m=[20 20 20]  v_m=[5 5 3]
  Display3 : Display
  Kdd : Constant  Value=Kdd
  Ktd : Constant  Value=Ktd
  Ktd2 : Constant  Value=densidadeAr
  Momentos de inercia : Constant  Value=IXYZ
  Scope1 : Scope  NumInputPorts=5
  Scope10 : Scope  NumInputPorts=3
  Scope2 : Scope  NumInputPorts=3
  Scope7 : Scope  NumInputPorts=3
  "area " : Constant  Value=areaLateral
  areaAsa : Constant  Value=areaAsa
  cdArrastoParasita : Constant  Value=cdArrastoParasita
  cdAviao : Constant  Value=cdAviao
  clAviao : Constant  Value=clAviao
  g : Constant  Value=g  SampleTime=sampleTime
  ib : Constant  Value=Lb
  kg : Constant  Value=massa  SampleTime=sampleTime
  st : Constant  Value=sampleTime
  XYZ : Outport
  XYZ_ponto : Outport  Port=2
  XYZ_ponto_ponto : Outport  Port=3
  phi_theta_psi : Outport  Port=4
  phi_theta_psi_ponto : Outport  Port=5
  wires:
  Dinâmica do sistema/1(estados) -> Delay1/1
  Delay1/1 -> Dinâmica do sistema/21(estados_anterior)
  ib/1 -> Dinâmica do sistema/15(lb)
  Momentos de inercia/1 -> Dinâmica do sistema/16(Ixyz)
  st/1 -> Dinâmica do sistema/20(dt)
  Kdd/1 -> Dinâmica do sistema/14(kdd)
  kg/1 -> Dinâmica do sistema/6(massaTotal)
  g/1 -> Dinâmica do sistema/5(gravidade)
  Ktd/1 -> Dinâmica do sistema/13(ktd)
  Dinâmica do sistema/5(XYZ) -> XYZ/1
  w3/1 -> Dinâmica do sistema/3(w3)
  w4/1 -> Dinâmica do sistema/4(w4)
  Dinâmica do sistema/6(XYZ_ponto) -> XYZ_ponto/1
  w2/1 -> Dinâmica do sistema/2(w2)
  Dinâmica do sistema/9(phi_theta_psi_ponto) -> phi_theta_psi_ponto/1
  Dinâmica do sistema/8(phi_theta_psi) -> phi_theta_psi/1
  w1/1 -> Dinâmica do sistema/1(w1)
  Dinâmica do sistema/2(U) -> Display3/1
  "area "/1 -> Dinâmica do sistema/8(areaAviao)
  cdArrastoParasita/1 -> Dinâmica do sistema/10(cdParasita)
  Ktd2/1 -> Dinâmica do sistema/7(rho)
  cdAviao/1 -> Dinâmica do sistema/11(cdAviao)
  clAviao/1 -> Dinâmica do sistema/12(clAviao)
  areaAsa/1 -> Dinâmica do sistema/9(areaAsa)
  Demux6/1 -> Scope7/1
  Demux6/2 -> Scope7/2
  Demux6/3 -> Scope7/3
  Dinâmica do sistema/14(arrastoTotal) -> Demux6/1
  beta/1 -> Dinâmica do sistema/18(beta)
  Dinâmica do sistema/10(thrustX) -> Demux1/1
  Dinâmica do sistema/11(arrastoParasita) -> Demux2/1
  Dinâmica do sistema/12(arrastoInduzido) -> Demux3/1
  Demux1/1 -> Add/1, Scope1/1  "motor frente"
  Demux2/1 -> Add/2, Scope1/2  "arrasto parasita"
  Demux3/1 -> Add/3, Scope1/3  "Arrasto induzido"
  Add/1 -> Scope1/4  "Total"
  Dinâmica do sistema/13(sustentacao) -> Demux5/1, Scope1/5  "sustentacao"
  Dinâmica do sistema/15(forcas) -> Demux4/1
  Demux4/3 -> Scope10/1  "motor"
  Demux5/3 -> Scope10/2  "sustentação"
  Dinâmica do sistema/16(gravidadeVec) -> Demux7/1
  Demux7/3 -> Scope10/3  "gravidade"
  Dinâmica do sistema/7(XYZ_ponto_ponto) -> XYZ_ponto_ponto/1
  Constant1/1 -> Dinâmica do sistema/17(velVento), Scope2/1
  alphaProfundor/1 -> Dinâmica do sistema/19(alphaProfundor)
  Constant/1 -> Discrete Wind Gust Model/1

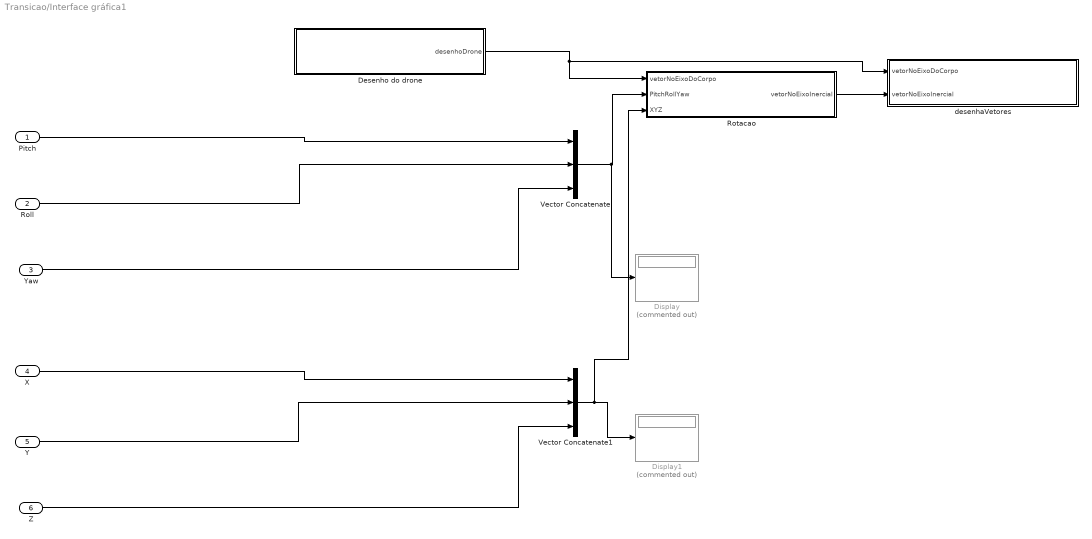
== system Transicao/Interface gráfica1 ==
  Pitch : Inport
  Roll : Inport  Port=2
  Yaw : Inport  Port=3
  X : Inport  Port=4
  Y : Inport  Port=5
  Z : Inport  Port=6
  Desenho do drone : MATLAB Function  TreatAsAtomicUnit=on
  Display : Display  Commented=on
  Display1 : Display  Commented=on
  Rotacao : MATLAB Function  TreatAsAtomicUnit=on
  Vector Concatenate : Concatenate  NumInputs=3
  Vector Concatenate1 : Concatenate  NumInputs=3
  desenhaVetores : MATLAB Function  TreatAsAtomicUnit=on
  wires:
  Roll/1 -> Vector Concatenate/2
  Z/1 -> Vector Concatenate1/3
  Y/1 -> Vector Concatenate1/2
  X/1 -> Vector Concatenate1/1
  Vector Concatenate/1 -> Rotacao/2(PitchRollYaw), Display/1
  Pitch/1 -> Vector Concatenate/1
  Yaw/1 -> Vector Concatenate/3
  Rotacao/1(vetorNoEixoInercial) -> desenhaVetores/2(vetorNoEixoInercial)
  Vector Concatenate1/1 -> Display1/1, Rotacao/3(XYZ)
  Desenho do drone/1(desenhoDrone) -> Rotacao/1(vetorNoEixoDoCorpo), desenhaVetores/1(vetorNoEixoDoCorpo)

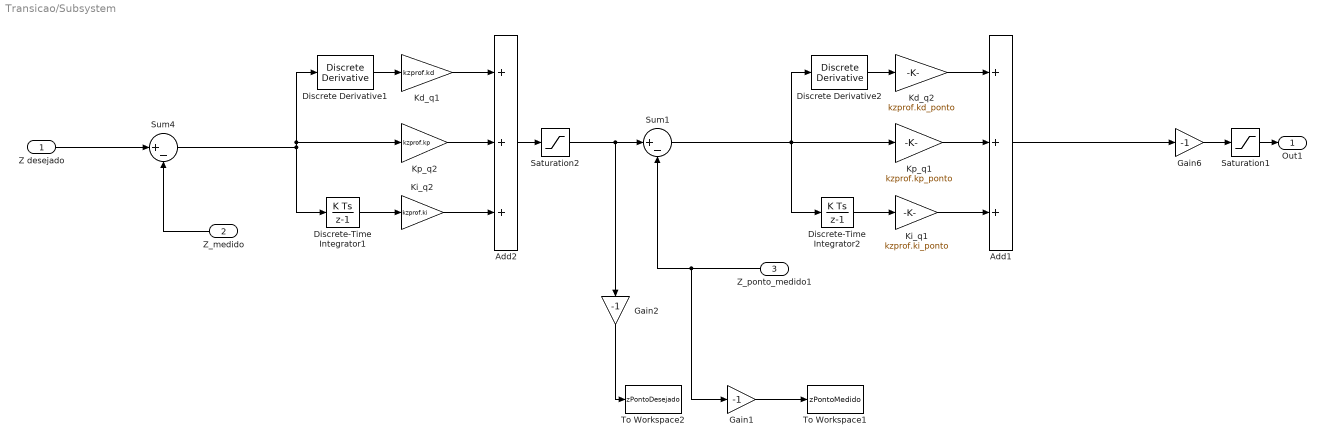
== system Transicao/Subsystem ==
  Z desejado : Inport
  Z_medido : Inport  Port=2
  Z_ponto_medido1 : Inport  Port=3
  Add1 : Sum  Inputs=+++
  Add2 : Sum  Inputs=+++
  Discrete Derivative1 : simulink/Discrete/Discrete Derivative  gainval=1.0  ICPrevScaledInput=0.0  InputProcessing=Inherited  OutMin=[]  OutMax=[]  OutDataType=fixdt(1, 16)  OutScaling=2^-10  DoSatur=off
  Discrete Derivative2 : simulink/Discrete/Discrete Derivative  gainval=1.0  ICPrevScaledInput=0.0  InputProcessing=Inherited  OutMin=[]  OutMax=[]  OutDataType=fixdt(1, 16)  OutScaling=2^-10  DoSatur=off
  Discrete-Time Integrator1 : DiscreteIntegrator  InitialConditionSetting=State (most efficient)  SampleTime=-1  ICPrevOutput=DiscIntNeverNeededParam  ICPrevScaledInput=DiscIntNeverNeededParam
  Discrete-Time Integrator2 : DiscreteIntegrator  InitialConditionSetting=State (most efficient)  SampleTime=-1  ICPrevOutput=DiscIntNeverNeededParam  ICPrevScaledInput=DiscIntNeverNeededParam
  Gain1 : Gain  Gain=-1
  Gain2 : Gain  Gain=-1
  Gain6 : Gain  Gain=-1
  Kd_q1 : Gain  Gain=kzprof.kd
  Kd_q2 : Gain  Gain=kzprof.kd_ponto
  Ki_q1 : Gain  Gain=kzprof.ki_ponto
  Ki_q2 : Gain  Gain=kzprof.ki
  Kp_q1 : Gain  Gain=kzprof.kp_ponto
  Kp_q2 : Gain  Gain=kzprof.kp
  Saturation1 : Saturate  UpperLimit=20*pi/180  LowerLimit=-20*pi/180  LinearizeAsGain=off
  Saturation2 : Saturate  UpperLimit=2  LowerLimit=-2  LinearizeAsGain=off
  Sum1 : Sum  Inputs=|+-
  Sum4 : Sum  Inputs=|+-
  To Workspace1 : ToWorkspace  VariableName=zPontoMedido  SaveFormat=Timeseries  SampleTime=-1
  To Workspace2 : ToWorkspace  VariableName=zPontoDesejado  SaveFormat=Timeseries  SampleTime=-1
  Out1 : Outport
  wires:
  Kd_q1/1 -> Add2/1
  Discrete-Time Integrator1/1 -> Ki_q2/1
  Discrete Derivative1/1 -> Kd_q1/1
  Saturation1/1 -> Out1/1
  Kp_q2/1 -> Add2/2
  Z desejado/1 -> Sum4/1
  Sum4/1 -> Discrete Derivative1/1, Kp_q2/1, Discrete-Time Integrator1/1
  Ki_q2/1 -> Add2/3
  Gain6/1 -> Saturation1/1
  Z_medido/1 -> Sum4/2
  Kd_q2/1 -> Add1/1
  Discrete-Time Integrator2/1 -> Ki_q1/1
  Discrete Derivative2/1 -> Kd_q2/1
  Kp_q1/1 -> Add1/2
  Sum1/1 -> Discrete Derivative2/1, Kp_q1/1, Discrete-Time Integrator2/1
  Ki_q1/1 -> Add1/3
  Add2/1 -> Saturation2/1
  Z_ponto_medido1/1 -> Gain1/1, Sum1/2
  Add1/1 -> Gain6/1
  Saturation2/1 -> Gain2/1, Sum1/1
  Gain1/1 -> To Workspace1/1
  Gain2/1 -> To Workspace2/1

== system Transicao/eta ==
  beta : Inport
  Constant : Constant  Value=pi/2
  Divide : Product  Inputs=*/
  eta : Outport
  wires:
  beta/1 -> Divide/1
  Divide/1 -> eta/1
  Constant/1 -> Divide/2

== matlab function Transicao/Atuador VC/Motor mixer ==
  data: u1thrust input; w1 output; u3mPitch input; w2 output; w3 output; w4 output; ktd input; kdd input; lb input; alphaProfundor output
% Transforma um comando de thrust e momento em velocidade angular
function [w1,w2,w3,w4, alphaProfundor]= fcn(u1thrust, u3mPitch, ktd, kdd, lb)
% Supondo que U seja força e momentos
%w2ParaU = [ Ktd      Ktd     Ktd      Ktd;
%          -Ktd*Lb   Ktd*Lb  Ktd*Lb  -Ktd*Lb;
%           Ktd*Lb  -Ktd*Lb  Ktd*Lb  -Ktd*Lb;
%          -Kdd     -Kdd     Kdd      Kdd]

w2ParaU = [ ktd      ktd     ktd      ktd;
           -ktd*lb(2)      ktd*lb(1)     ktd*lb(1)     -ktd*lb(2);
            ktd*lb(3)     -ktd*lb(4)     ktd*lb(3)     -ktd*lb(4);
           -kdd     -kdd       kdd      kdd];


w = inv(w2ParaU)*[u1thrust ; 0 ; 0 ; 0];
alphaProfundor = u3mPitch;
for i = 1:numel(w);
   if(w(i) > 500.75^2)
      w(i) = 500.75^2; 
   end
end
for i = 1:numel(w);
   if(w(i) < 0)
      w(i) = 0; 
   end
end

w1 = sqrt(w(1));
w2 = 0;
w3 = sqrt(w(3));
w4 = 0;
